simulink model "test20"  (R2021a)
settings: Solver=ode23tb  StartTime=0.0  StopTime=10  RelTol=1e-3
model workspace (MAT data in the model file):
  params = climate_p
  params.H = 7.99977069808
  params.A_f = 3100.00026794
  params.A_c = 3299.99999958
  params.minWindows = 0.49999998574
  params.alpha_i = 0.0143839885631
  params.cd_c = 8999.32112543
  params.T_ss = 285
values from neighbouring files (symbols this model uses):
  beta = 2.0    (= 2)    [test20_script.m]
  gamma = 0.01    [test20_script.m]
undefined symbols (not defined in the file or in its folder): AR
libraries: HORTISIM x5
settings Model: OrderedModelArguments=off  Creator=djoroya  LastModifiedBy=djoroya
settings DebuggingCC: UnconnectedInputMsg=none  UnconnectedOutputMsg=none  UnconnectedLineMsg=none

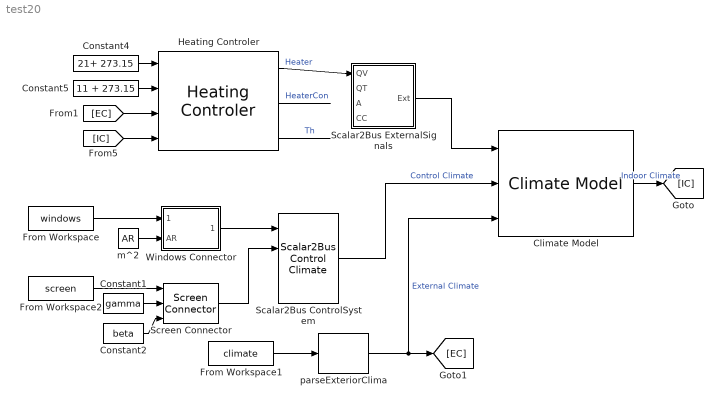
== system test20 ==
  Climate Model : HORTISIM/Climate/Models/Climate Model  params=climate_params  x0=cic
      settings: SourceProductName=Horti Simulator
  Constant1 : Constant  Value=gamma
  Constant2 : Constant  Value=beta
  Constant4 : Constant  Value=21+ 273.15
  Constant5 : Constant  Value=11 + 273.15
  From Workspace : FromWorkspace  VariableName=windows
  From Workspace1 : FromWorkspace  VariableName=climate
  From Workspace2 : FromWorkspace  VariableName=screen
  Heating Controler : HORTISIM/Climate/Controls/Heating Controler  params=heat_p  x0=heat_ic
      settings: SourceProductName=Horti Simulator
  Scalar2Bus ControlSystem : HORTISIM/Other  Functions/Scalar2Bus  Control Climate  SystemSampleTime=-1  VariantActivationTime=update diagram  Latency=0  AutoFrameSizeCalculation=off
      settings: SourceProductName=Horti Simulator
  Scalar2Bus ExternalSignals : Subsystem
  "Screen Connector " : HORTISIM/Other  Functions/Screen Connector  SystemSampleTime=-1  VariantActivationTime=update diagram  Latency=0  AutoFrameSizeCalculation=off
      settings: SourceProductName=Horti Simulator
  Windows Connector : Subsystem
  m^2 : Constant  Value=AR
  "parseExteriorClima " : HORTISIM/Other  Functions/parseExteriorClima  SystemSampleTime=-1  VariantActivationTime=update diagram  Latency=0  AutoFrameSizeCalculation=off
      settings: SourceProductName=Horti Simulator
  wires:
  Windows Connector/1(Windows) -> Scalar2Bus ControlSystem/1
  m^2/1 -> Windows Connector/2(AR)
  From Workspace/1 -> Windows Connector/1(value)
  "Screen Connector "/1 -> Scalar2Bus ControlSystem/2
  Climate Model/1 -> [IC]  "Indoor Climate"
  Scalar2Bus ControlSystem/1 -> Climate Model/2  "Control Climate"
  From Workspace1/1 -> "parseExteriorClima "/1
  "parseExteriorClima "/1 -> [EC], Climate Model/3  "External Climate"
  Constant2/1 -> "Screen Connector "/3
  Constant1/1 -> "Screen Connector "/2
  From Workspace2/1 -> "Screen Connector "/1
  Heating Controler/2 -> ?  "HeaterCon"
  Constant4/1 -> Heating Controler/1
  Heating Controler/3 -> ?  "Th"
  Heating Controler/1 -> Scalar2Bus ExternalSignals/1(QV)  "Heater"
  [IC] -> Heating Controler/4
  [EC] -> Heating Controler/3
  Constant5/1 -> Heating Controler/2
  Scalar2Bus ExternalSignals/1(Ext) -> Climate Model/1

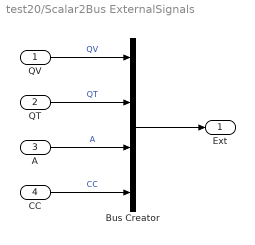
== system test20/Scalar2Bus ExternalSignals ==
  QV : Inport
  QT : Inport  Port=2
  A : Inport  Port=3
  CC : Inport  Port=4
  Bus Creator : BusCreator  Inputs=4
  Ext : Outport
  wires:
  QT/1 -> Bus Creator/2  "QT"
  QV/1 -> Bus Creator/1  "QV"
  A/1 -> Bus Creator/3  "A"
  CC/1 -> Bus Creator/4  "CC"
  Bus Creator/1 -> Ext/1

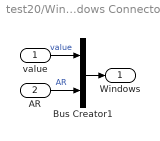
== system test20/Windows Connector ==
  value : Inport
  AR : Inport  Port=2
  Bus Creator1 : BusCreator  Inputs=2
  Windows : Outport
  wires:
  Bus Creator1/1 -> Windows/1
  value/1 -> Bus Creator1/1  "value"
  AR/1 -> Bus Creator1/2  "AR"
